simulink model "DLC_2a"  (R2023a)
settings: Solver=ode4  StartTime=0.0  StopTime=40  FixedStep=0.005  RelTol=1e-3
InitFcn:
  | DLC2
values from neighbouring files (symbols this model uses):
  K_scheduled = zeros(length(V_op), 2)    [CAL3.m]    (also in CUB.m; DLC2.m; MUS.m; OHZ.m)
  V_op = 5:5:85    [CAL3.m]    (also in CUB.m; DLC2.m; MUS.m; OHZ.m)
  X_track = [linspace(0, runway_length, 200)'; runway_length + R_track * cos(theta_circ(2:end))]    [CAL3.m]    (also in CUB.m = [0; 5000]; DLC2.m = 0:0.1:total_track_length; MUS.m = [0; 2000]; OHZ.m = [0; 2000])
  Y_track = [zeros(200, 1); R_track + R_track * sin(theta_circ(2:end))]    [CAL3.m]    (also in CUB.m = [0; 0]; DLC2.m = zeros(size(X_track)); MUS.m = [0; 0]; OHZ.m = [0; 0])
undefined symbols (not defined in the file or in its folder): planner_params, track_params, veh_params
libraries: simulink x2, slpidlib x2
(part 2 of 3)

== matlab function DLC_2a/Scopes/MATLAB Function1 ==
  settings: updateMethod=DISCRETE
  data: delta input; psi input; psi_ref input; Fx input; Fy input; Fz input; Trl input; Trr input; Tf_f input; Trl_f input; Trr_f input; w_vec input; vx input; vy input; ax input; ay input
function vehicle_frame_plotter(delta, psi, psi_ref, Fx, Fy, Fz, Trl, Trr, Tf_f, Trl_f, Trr_f, w_vec, vx, vy, ax, ay)
    coder.extrinsic('figure', 'plot', 'hold', 'axis', 'title', 'set', 'drawnow', 'patch', 'text', 'line', 'quiver', 'sprintf');
    
    persistent hWheels hSteer hSpokes hPsiRef hPsiAct hFlags hTqFlags hMotors hAxleFront hCircles hGdots hSwLabel hRwLabel hAngleLabel hVelArrow hAccArrow hVelText hAccText hCrosshairs counter
    
    if isempty(counter)
        % =====================================================================
        % STRICT CODER INITIALIZATION
        % =====================================================================
        counter = 0;
        hSteer = 0.0; hPsiRef = 0.0; hPsiAct = 0.0; hAxleFront = 0.0;
        hWheels = zeros(1,4); hFlags = zeros(1,4); hTqFlags = zeros(1,2); hMotors = zeros(1,2);
        hSpokes = zeros(1,3); hCircles = zeros(1,4); hGdots = zeros(1,4);
        hSwLabel = 0.0; hRwLabel = 0.0; hAngleLabel = 0.0;
        hVelArrow = 0.0; hAccArrow = 0.0; hVelText = 0.0; hAccText = 0.0;
        hCrosshairs = zeros(1,2);
        
        figure('Name', 'Vehicle Frame Telemetry - Car A', 'Color', 'w', 'Position', [100, 100, 750, 750]);
        hold on;
        
        % Chassis Outline & Front Axle
        plot([-1, 1, 1, -1, -1], [2, 2, -2, -2, 2], 'k', 'LineWidth', 2);
        hAxleFront = double(line([1, -1], [1.5, 1.5], 'Color', [0.2 0.2 0.2], 'LineWidth', 2));
        
        % Wheels Array Setup [FL, FR, RL, RR]
        for i = 1:4; hWheels(i) = double(patch(0, 0, [0.3 0.3 0.3])); end
        
        % =====================================================================
        % FRICTION CIRCLES, STEERING WHEEL, & YAW VECTORS
        % =====================================================================
        th_c = 0:0.1:2*pi;
        circle_x = cos(th_c); circle_y = sin(th_c);
        c_pos = [-2.0, 2.3; 2.0, 2.3; -2.0, -2.3; 2.0, -2.3]; 
        for i = 1:4
            hCircles(i) = double(plot(c_pos(i,1) + 0.5*circle_x, c_pos(i,2) + 0.5*circle_y, 'Color', [0.6 0 0.6], 'LineStyle', '--', 'LineWidth', 1.2));
            hGdots(i) = double(plot(c_pos(i,1), c_pos(i,2), 'mo', 'MarkerFaceColor', 'm', 'MarkerSize', 5));
        end
        
        hSteer = double(plot(0.4*cos(th_c), 0.4*sin(th_c) + 0.5, 'k', 'LineWidth', 3));
        hSpokes(1) = double(line([0, 0], [0.5, 0.5], 'Color', 'k', 'LineWidth', 2.5));
        hSpokes(2) = double(line([0, 0], [0.5, 0.5], 'Color', 'k', 'LineWidth', 2.5));
        hSpokes(3) = double(line([0, 0], [0.5, 0.5], 'Color', 'k', 'LineWidth', 2.5));
        
        hPsiRef = double(quiver(0, 1.8, 0, 0.8, 'r', 'LineWidth', 2.5, 'MaxHeadSize', 2));
        hPsiAct = double(quiver(0, 1.8, 0, 0.8, 'b', 'LineWidth', 2.5, 'MaxHeadSize', 2));
        
        for i = 1:4; hFlags(i) = double(text(0, 0, '', 'FontSize', 8, 'BackgroundColor', [1 1 1 0.8], 'EdgeColor', 'k')); end
        
        % =====================================================================
        % VEHICLE A POWERTRAIN GRAPHIC (Dual Motors)
        % =====================================================================
        m_b = [-.15, .15, .15, -.15]; m_w = [.2, .2, -.2, -.2];
        hMotors(1) = double(patch(m_b - 0.6, m_w - 1.5, [0.5 0.5 0.5])); % Left Motor
        hMotors(2) = double(patch(m_b + 0.6, m_w - 1.5, [0.5 0.5 0.5])); % Right Motor
        
        hTqFlags(1) = double(text(-0.6, -0.9, '', 'FontSize', 10, 'FontWeight', 'bold', 'HorizontalAlignment', 'center'));
        hTqFlags(2) = double(text(0.6, -0.9, '', 'FontSize', 10, 'FontWeight', 'bold', 'HorizontalAlignment', 'center'));
        
        % Labels
        hSwLabel = double(text(0, 1.2, '', 'FontSize', 9, 'FontWeight', 'bold', 'HorizontalAlignment', 'center'));
        hRwLabel = double(text(0, 1.65, '', 'FontSize', 9, 'FontWeight', 'bold', 'HorizontalAlignment', 'center', 'Color', [0 0.5 0]));
        hAngleLabel = double(text(0, 2.8, '', 'FontSize', 10, 'FontWeight', 'bold', 'HorizontalAlignment', 'center', 'Color', [0.4 0 0.6]));

        % =====================================================================
        % SHARED-ORIGIN VELOCITY & ACCELERATION VECTORS
        % =====================================================================
        hCrosshairs(1) = double(plot([-2.0 2.0], [-3.8 -3.8], 'k:', 'Color', [0.7 0.7 0.7]));
        hCrosshairs(2) = double(plot([0 0], [-4.2 -1.8], 'k:', 'Color', [0.7 0.7 0.7]));

        hVelArrow = double(quiver(0, -3.8, 0, 0, 'Color', [0 0.4 0.8], 'LineWidth', 2.5, 'MaxHeadSize', 2, 'AutoScale', 'off'));
        hAccArrow = double(quiver(0, -3.8, 0, 0, 'Color', [0.8 0.3 0], 'LineWidth', 2.5, 'MaxHeadSize', 2, 'AutoScale', 'off'));

        hVelText = double(text(-2.0, -4.3, '', 'FontSize', 9, 'FontWeight', 'bold', 'HorizontalAlignment', 'center', 'Color', [0 0.4 0.8]));
        hAccText = double(text(2.0, -4.3, '', 'FontSize', 9, 'FontWeight', 'bold', 'HorizontalAlignment', 'center', 'Color', [0.8 0.3 0]));
        
        axis([-4.5 4.5 -4.5 4.5]); axis equal; grid on;
        title('Dynamics - Car A (Dual Motor): Forces & Friction Circles');
    end
    counter = counter + 1;
    
    % --- UPDATE LOOP ---
    if mod(counter, 10) == 0
        R_delta = [cos(delta) -sin(delta); sin(delta) cos(delta)];
        w_orig = [-.2 .2 .2 -.2; .4 .4 -.4 -.4]; 
        w_rot = R_delta * w_orig;
        
        set(hWheels(1), 'XData', w_rot(1,:) - 1, 'YData', w_rot(2,:) + 1.5); 
        set(hWheels(2), 'XData', w_rot(1,:) + 1, 'YData', w_rot(2,:) + 1.5); 
        set(hWheels(3), 'XData', w_orig(1,:) - 1, 'YData', w_orig(2,:) - 1.5); 
        set(hWheels(4), 'XData', w_orig(1,:) + 1, 'YData', w_orig(2,:) - 1.5); 
        
        set(hAxleFront, 'XData', [mean(w_rot(1,:) - 1), mean(w_rot(1,:) + 1)], 'YData', [mean(w_rot(2,:) + 1.5), mean(w_rot(2,:) + 1.5)]);
        
        sw_a = delta * 14; 
        th_sw = (0:0.1:2*pi) + sw_a;
        set(hSteer, 'XData', 0.4*cos(th_sw), 'YData', 0.4*sin(th_sw) + 0.5);
        spk = [0, pi, 1.5*pi] + sw_a;
        for j=1:3; set(hSpokes(j), 'XData', [0, 0.4*cos(spk(j))], 'YData', [0.5, 0.5 + 0.4*sin(spk(j))]); end
        
        set(hSwLabel, 'String', sprintf('SW: %.1f deg', sw_a * 180/pi));
        set(hRwLabel, 'String', sprintf('RW: %.1f deg', delta * 180/pi));
        
        psi_e = psi_ref - psi; 
        set(hPsiRef, 'UData', 0.8*sin(psi_e), 'VData', 0.8*cos(psi_e));
        set(hPsiAct, 'UData', 0, 'VData', 0.8);
        set(hAngleLabel, 'String', sprintf('Sideslip: %.1f deg', psi_e * 180/pi));
        
        fb = [abs(Tf_f/2), abs(Tf_f/2), abs(Trl_f), abs(Trr_f)]; 
        mu = 1.0;
        c_pos = [-2.0, 2.3; 2.0, 2.3; -2.0, -2.3; 2.0, -2.3]; 
        th_c = 0:0.1:2*pi;
        rpm_vec = w_vec * (30 / pi);
        
        for i = 1:4
            if fb(i) > 5; set(hWheels(i), 'FaceColor', [0.8 0 0]); else set(hWheels(i), 'FaceColor', [0.3 0.3 0.3]); end
            F_max = max(100, mu * Fz(i));
            scale = 0.5 / 6000; 
            set(hCircles(i), 'XData', c_pos(i,1) + F_max*scale*cos(th_c), 'YData', c_pos(i,2) + F_max*scale*sin(th_c));
            set(hGdots(i), 'XData', c_pos(i,1) + Fy(i)*scale, 'YData', c_pos(i,2) + Fx(i)*scale);
        end
        
        % Dual Motor Visualization Logic
        mt = [Trl, Trr]; 
        for k = 1:2
            if mt(k) > 0.1; set(hMotors(k), 'FaceColor', [0 0.7 0]); 
            elseif mt(k) < -0.1; set(hMotors(k), 'FaceColor', [0.7 0 0]); 
            else set(hMotors(k), 'FaceColor', [0.5 0.5 0.5]); end
            
            set(hTqFlags(k), 'String', sprintf('%.1f Nm', mt(k)));
        end
        
        pos = [-4.1, 1.5; 2.8, 1.5; -4.1, -1.5; 2.8, -1.5]; 
        for i = 1:4
            f_str = sprintf('Fx: %.0f\nFy: %.0f\nFz: %.0f\nFric: %.1f\nRPM: %.0f', Fx(i), Fy(i), Fz(i), fb(i), rpm_vec(i));
            set(hFlags(i), 'Position', [pos(i,1), pos(i,2)], 'String', f_str);
        end

        % =====================================================================
        % UPDATE DYNAMIC VECTORS
        % =====================================================================
        vx_kmh = vx * 3.6;
        vy_kmh = vy * 3.6;
        ax_g = ax / 9.81;
        ay_g = ay / 9.81;

        vel_scale = 0.015; 
        acc_scale = 0.8;   

        set(hVelArrow, 'UData', -vy_kmh * vel_scale, 'VData', vx_kmh * vel_scale);
        set(hAccArrow, 'UData', -ay_g * acc_scale, 'VData', ax_g * acc_scale);

        set(hVelText, 'String', sprintf('Vx: %.1f | Vy: %.1f\n[km/h]', vx_kmh, vy_kmh));
        set(hAccText, 'String', sprintf('Ax: %.2f | Ay: %.2f\n[G]', ax_g, ay_g));
        
        drawnow limitrate;
    end
end

== matlab function DLC_2a/Vehicle & Powertrain Plant1/MATLAB Function ==
  data: delta input; Trr_m input; Trl_m input; Trr_f input; Trl_f input; Tf_f input; vx input; vy input; r input; psi input; SOC input; T_batt input; T_motor input; w_fl input; w_fr input; w_rl input; w_rr input; vx_dot output; vy_dot output; r_dot output; X_dot output; Y_dot output; psi_dot output; s_dot output; SOC_dot output; T_batt_dot output; T_mot_dot output; Fz_f_tot output; Fz_r_tot output; Fz_rl output; Fz_rr output; Fx_vec output; Fy_vec output; Fz_vec output; w_vec output; w_dot_vec output; veh_params parameter
function [vx_dot, vy_dot, r_dot, X_dot, Y_dot, psi_dot, s_dot, SOC_dot, T_batt_dot, T_mot_dot, Fz_f_tot, Fz_r_tot, Fz_rl, Fz_rr, Fx_vec, Fy_vec, Fz_vec, w_vec, w_dot_vec] = vehicle_physics_engine(delta, Trr_m, Trl_m, Trr_f, Trl_f, Tf_f, vx, vy, r, psi, SOC, T_batt, T_motor, w_fl, w_fr, w_rl, w_rr, veh_params)
    % =========================================================================
    % HIGH-FIDELITY EV VEHICLE DYNAMICS PLANT MODEL (ANTI-SINGULARITY PATCHED)
    % =========================================================================
    
    % ---------------------------------------------------------------------
    % 1. UNPACK CENTRALIZED PARAMETERS
    % ---------------------------------------------------------------------
    m = veh_params.m; Iz = veh_params.Iz; lf = veh_params.lf; lr = veh_params.lr; L = veh_params.L;
    tw = veh_params.tw; h_cg = veh_params.h_cg; Rw = veh_params.Rw; Iw = veh_params.Iw; 
    G = veh_params.G; g = veh_params.g; rho = veh_params.rho; CdA = veh_params.CdA;
    roll_bias_f = veh_params.roll_bias_f; 
    
    mu_max = veh_params.mu_max; C_rr = veh_params.C_rr;
    ks_f = veh_params.ks_f; ks_r = veh_params.ks_r;
    C_tire = veh_params.C_tire; E_tire = veh_params.E_tire;
    
    if abs(vx) < 0.5
        vx_safe = 0.5 * sign(vx + 1e-6); % Prevents absolute zero, preserves direction
    else
        vx_safe = vx;
    end
    
    % FIX 1: Preserved-Sign Aerodynamic Drag
    % vx_safe * abs(vx_safe) ensures drag always pushes AGAINST the car, even in reverse.
    F_aero_drag = 0.5 * rho * CdA * vx_safe * abs(vx_safe);

    % ---------------------------------------------------------------------
    % 2. DYNAMIC TIRE PEAK CALIBRATION
    % ---------------------------------------------------------------------
    Fz_axle_f_static = m * g * (lr / L); 
    Fz_axle_r_static = m * g * (lf / L); 
    
    D_tire_f = mu_max * (Fz_axle_f_static / 2); 
    D_tire_r = mu_max * (Fz_axle_r_static / 2); 
    
    B_tire_f = ks_f / (C_tire * D_tire_f * 2); 
    B_tire_r = ks_r / (C_tire * D_tire_r * 2); 
    
    % ---------------------------------------------------------------------
    % 3. 3D WEIGHT TRANSFER (WITH SUSPENSION CAPS)
    % ---------------------------------------------------------------------
    Trr_tot = Trr_m * G + Trr_f;
    Trl_tot = Trl_m * G + Trl_f;
    Tf_tot_half = Tf_f / 2; 
    
    Fx_fl_tq = Tf_tot_half / Rw; Fx_fr_tq = Tf_tot_half / Rw;
    Fx_rl_tq = Trl_tot / Rw; Fx_rr_tq = Trr_tot / Rw;
    
    % Using corrected aero drag
    ax_est = ((Fx_fl_tq + Fx_fr_tq + Fx_rl_tq + Fx_rr_tq) - F_aero_drag) / m;
    ay_est = vx_safe * r;
    
    Fz_f_tot = m * g * (lr / L) - m * ax_est * (h_cg / L);
    Fz_r_tot = m * g * (lf / L) + m * ax_est * (h_cg / L);
    
    dFz_y_f = m * ay_est * (h_cg / tw) * roll_bias_f;
    dFz_y_r = m * ay_est * (h_cg / tw) * (1 - roll_bias_f);
    
    % FIX 2: Suspension Caps. Prevents Fz from exceeding physical limits in a spin
    Fz_max_f = Fz_axle_f_static * 2.5; 
    Fz_max_r = Fz_axle_r_static * 2.5;
    
    Fz_fl = max(100, min(Fz_max_f, Fz_f_tot / 2 + dFz_y_f));
    Fz_fr = max(100, min(Fz_max_f, Fz_f_tot / 2 - dFz_y_f));
    Fz_rl = max(100, min(Fz_max_r, Fz_r_tot / 2 + dFz_y_r));
    Fz_rr = max(100, min(Fz_max_r, Fz_r_tot / 2 - dFz_y_r));
    Fz_vec = [Fz_fl, Fz_fr, Fz_rl, Fz_rr];
    
    % ---------------------------------------------------------------------
    % 4. VECTOR-SUM PACEJKA COMBINED SLIP MODEL
    % ---------------------------------------------------------------------
    v_hub_fl = vx_safe - (tw / 2) * r; v_hub_fr = vx_safe + (tw / 2) * r;
    v_hub_rl = vx_safe - (tw / 2) * r; v_hub_rr = vx_safe + (tw / 2) * r;
    
    k_fl = (w_fl * Rw - v_hub_fl) / max(abs(v_hub_fl), 1.0);
    k_fr = (w_fr * Rw - v_hub_fr) / max(abs(v_hub_fr), 1.0);
    k_rl = (w_rl * Rw - v_hub_rl) / max(abs(v_hub_rl), 1.0);
    k_rr = (w_rr * Rw - v_hub_rr) / max(abs(v_hub_rr), 1.0);
    
    % FIX 3: Absolute value on denomiator prevents inverted slip angles in reverse
    alpha_fl = delta - atan((vy + lf * r) / max(abs(v_hub_fl), 1.0));
    alpha_fr = delta - atan((vy + lf * r) / max(abs(v_hub_fr), 1.0));
    alpha_rl = -atan((vy - lr * r) / max(abs(v_hub_rl), 1.0));
    alpha_rr = -atan((vy - lr * r) / max(abs(v_hub_rr), 1.0));
    
    sigma_fl = sqrt(k_fl^2 + tan(alpha_fl)^2) + 1e-6;
    sigma_fr = sqrt(k_fr^2 + tan(alpha_fr)^2) + 1e-6;
    sigma_rl = sqrt(k_rl^2 + tan(alpha_rl)^2) + 1e-6;
    sigma_rr = sqrt(k_rr^2 + tan(alpha_rr)^2) + 1e-6;
    
    F_tot_fl = mu_max * Fz_fl * sin(C_tire * atan(B_tire_f * sigma_fl - E_tire * (B_tire_f * sigma_fl - atan(B_tire_f * sigma_fl))));
    F_tot_fr = mu_max * Fz_fr * sin(C_tire * atan(B_tire_f * sigma_fr - E_tire * (B_tire_f * sigma_fr - atan(B_tire_f * sigma_fr))));
    F_tot_rl = mu_max * Fz_rl * sin(C_tire * atan(B_tire_r * sigma_rl - E_tire * (B_tire_r * sigma_rl - atan(B_tire_r * sigma_rl))));
    F_tot_rr = mu_max * Fz_rr * sin(C_tire * atan(B_tire_r * sigma_rr - E_tire * (B_tire_r * sigma_rr - atan(B_tire_r * sigma_rr))));
    
    Fx_fl = F_tot_fl * (k_fl / sigma_fl) - C_rr * Fz_fl * tanh(v_hub_fl * 10);
    Fx_fr = F_tot_fr * (k_fr / sigma_fr) - C_rr * Fz_fr * tanh(v_hub_fr * 10);
    Fx_rl = F_tot_rl * (k_rl / sigma_rl) - C_rr * Fz_rl * tanh(v_hub_rl * 10);
    Fx_rr = F_tot_rr * (k_rr / sigma_rr) - C_rr * Fz_rr * tanh(v_hub_rr * 10);
    Fx_vec = [Fx_fl, Fx_fr, Fx_rl, Fx_rr];
    
    Fy_fl = F_tot_fl * (tan(alpha_fl) / sigma_fl);
    Fy_fr = F_tot_fr * (tan(alpha_fr) / sigma_fr);
    Fy_rl = F_tot_rl * (tan(alpha_rl) / sigma_rl);
    Fy_rr = F_tot_rr * (tan(alpha_rr) / sigma_rr);
    Fy_vec = [Fy_fl, Fy_fr, Fy_rl, Fy_rr];
    
    % ---------------------------------------------------------------------
    % 5. CHASSIS & WHEEL INTEGRATORS
    % ---------------------------------------------------------------------
    w_fl_dot = (-abs(Tf_f / 2) * sign(w_fl) - Fx_fl * Rw) / Iw;
    w_fr_dot = (-abs(Tf_f / 2) * sign(w_fr) - Fx_fr * Rw) / Iw;
    w_rl_dot = (Trl_m * G - abs(Trl_f) * sign(w_rl) - Fx_rl * Rw) / Iw;
    w_rr_dot = (Trr_m * G - abs(Trr_f) * sign(w_rr) - Fx_rr * Rw) / Iw;
    w_dot_vec = [w_fl_dot, w_fr_dot, w_rl_dot, w_rr_dot];
    w_vec = [w_fl, w_fr, w_rl, w_rr];
    
    sum_Fx = (Fx_fl + Fx_fr) * cos(delta) - (Fy_fl + Fy_fr) * sin(delta) + Fx_rl + Fx_rr;
    vx_dot = (sum_Fx - F_aero_drag) / m + vy * r;
    
    sum_Fy = (Fy_fl + Fy_fr) * cos(delta) + (Fx_fl + Fx_fr) * sin(delta) + Fy_rl + Fy_rr;
    vy_dot = sum_Fy / m - vx_safe * r;
    
    M_front = lf * ((Fy_fl + Fy_fr) * cos(delta) + (Fx_fl + Fx_fr) * sin(delta));
    M_rear  = -lr * (Fy_rl + Fy_rr);
    M_tv    = (Fx_rr - Fx_rl) * (tw / 2); 
    r_dot  = (M_front + M_rear + M_tv) / Iz;
    
    X_dot   = vx_safe * cos(psi) - vy * sin(psi);
    Y_dot   = vx_safe * sin(psi) + vy * cos(psi);
    psi_dot = r;
    s_dot   = vx_safe;
    
    % ---------------------------------------------------------------------
    % 6. THERMALS & SOC
    % ---------------------------------------------------------------------
    P_mech = (Trr_m + Trl_m) * G * (vx_safe / Rw);
    P_elec = P_mech; 
    
    if P_mech > 500
        P_elec = P_mech / 0.90; 
    elseif P_mech < -500
        P_elec = P_mech * 0.90; 
    end
    
    I_curr = P_elec / veh_params.V_pack;
    SOC_dot = -I_curr / (veh_params.Cap_Ah * 3600);
    
    T_batt_dot = ((I_curr^2) * veh_params.R_pack - veh_params.hA_cool_batt * (T_batt - veh_params.T_coolant_batt)) / (veh_params.m_batt * veh_params.cp_batt);
    T_mot_dot  = (abs(P_elec - P_mech) - veh_params.hA_cool_motor * (T_motor - veh_params.T_ambient)) / (veh_params.m_motor * veh_params.cp_motor);
end

== matlab function DLC_2a/Vehicle Control Unit (VCU)1/MATLAB Function ==
  data: delta_curr input; pedal input; T_rr_motor_raw output; vx_curr input; vy_curr input; r_curr input; kappa_ref input; Fz_f_total input; Fz_r_total input; Fz_rl input; Fz_rr input; SOC input; T_batt input; T_motor input; V_op parameter; K_scheduled parameter; T_rl_motor_raw output; T_rr_fric output; w_vec input; T_rl_fric output; T_f_fric output; Mz_cmd output; r_ref output
function [T_rr_motor_raw, T_rl_motor_raw, T_rr_fric, T_rl_fric, T_f_fric, Mz_cmd, r_ref] = vcu_allocator(delta_curr, pedal, vx_curr, vy_curr, r_curr, kappa_ref, Fz_f_total, Fz_r_total, Fz_rl, Fz_rr, SOC, T_batt, T_motor, V_op, K_scheduled, w_vec)
    
    T_rr_motor_raw = 0.0;
    T_rl_motor_raw = 0.0;
    T_rr_fric = 0.0;
    T_rl_fric = 0.0;
    T_f_fric = 0.0;
    Mz_cmd = 0.0;
    Rw = 0.34; tw = 1.65; G = 10; mu_max = 1.2;
    
    % --- Per-Motor Limits (Total System = 500 kW, 800 Nm) ---
    P_motor_base = 250000; % 250 kW per motor 
    T_motor_max = 400;     % 400 Nm per motor 
    T_fric_max_per_wheel = 3500;
    % --------------------------------------------------------
    
    % --- Battery and Thermal Derating ---
    T_batt_cal = [-10, 0, 15, 45, 55, 60]; P_derate_batt_cal = [0, 0.5, 1.0, 1.0, 0.2, 0];
    T_motor_cal = [30, 90, 110, 130, 150]; P_derate_motor_cal = [1.0, 1.0, 0.8, 0.2, 0];
    SOC_vec = [0, 0.05, 0.15, 0.85, 0.95, 1.0]; 
    P_derate_SOC_dis = [0, 0.1, 1.0, 1.0, 1.0, 1.0]; P_derate_SOC_chg = [1.0, 1.0, 1.0, 1.0, 0.1, 0];
    
    derate_T_batt = interp1(T_batt_cal, P_derate_batt_cal, T_batt(1), 'linear', 0);
    derate_T_mot  = interp1(T_motor_cal, P_derate_motor_cal, T_motor(1), 'linear', 0);
    derate_T_total = min(derate_T_batt, derate_T_mot);
    
    derate_S_dis = interp1(SOC_vec, P_derate_SOC_dis, SOC(1), 'linear', 0);
    derate_S_chg = interp1(SOC_vec, P_derate_SOC_chg, SOC(1), 'linear', 0);
    
    P_avail_dis = P_motor_base * min(derate_T_total, derate_S_dis);
    P_avail_chg = P_motor_base * min(derate_T_total, derate_S_chg);
    
    vx_lqr = max(vx_curr(1), 5.0);
    
    % --- Speed-based Torque Vectoring Blending (45 km/h to 50 km/h) ---
    vx_kmh = vx_curr(1) * 3.6;
    tv_blend_lower = 45.0; 
    tv_blend_upper = 50.0; 
    
    if vx_kmh >= tv_blend_upper
        tv_blend = 1.0;
    elseif vx_kmh <= tv_blend_lower
        tv_blend = 0.0;
    else
        tv_blend = (vx_kmh - tv_blend_lower) / (tv_blend_upper - tv_blend_lower);
    end
    
    % --- LQR Yaw Moment Calculation ---
    K_dyn_1 = interp1(V_op, K_scheduled(:,1), vx_lqr, 'linear', 'extrap');
    K_dyn_2 = interp1(V_op, K_scheduled(:,2), vx_lqr, 'linear', 'extrap');
             
    % Dynamic Ackermann Reference
    L = 2.6; % Wheelbase
    K_us = 0.002; % Small understeer gradient (optional)
    r_ref = (vx_lqr * delta_curr(1)) / (L * (1 + K_us * vx_lqr^2));
    
    Mz_req = tv_blend * -(K_dyn_1(1) * vy_curr(1) + K_dyn_2(1) * (r_curr(1) - r_ref));
    Mz_cmd = max(-2500, min(2500, Mz_req)); 
    
    T_delta_wheel_raw = max(-1500, min(1500, (Mz_cmd * Rw) / tw));
    
    % =========================================================================
    % --- DYNAMIC MOTOR POWER LIMITS (Hyperbolic Torque Derating) ---
    % =========================================================================
    % Calculate actual motor speed from wheel speed (rad/s)
    % w_vec = [w_fl, w_fr, w_rl, w_rr]
    w_motor_rl = max(abs(w_vec(3) * G), 0.1); % Prevent div-by-zero at standstill
    w_motor_rr = max(abs(w_vec(4) * G), 0.1); 
    
    % Power-limited torque curve: T_max = P_max / w
    T_limit_rl_dis = P_avail_dis / w_motor_rl;
    T_limit_rr_dis = P_avail_dis / w_motor_rr;
    T_limit_rl_chg = P_avail_chg / w_motor_rl;
    T_limit_rr_chg = P_avail_chg / w_motor_rr;
    
    % Final motor bounds (Minimum of Inverter current limit and Power limit)
    T_motor_lim_rl_dis = min(T_motor_max, T_limit_rl_dis);
    T_motor_lim_rr_dis = min(T_motor_max, T_limit_rr_dis);
    
    T_motor_lim_rl_chg = max(-T_motor_max, -T_limit_rl_chg);
    T_motor_lim_rr_chg = max(-T_motor_max, -T_limit_rr_chg);
    % =========================================================================
    
    T_grip_lim_rl_wheel = mu_max * Fz_rl(1) * Rw * 0.90; 
    T_grip_lim_rr_wheel = mu_max * Fz_rr(1) * Rw * 0.90;
    
    % Combine physical motor limits with dynamic grip limits
    T_max_rl_motor = min(T_motor_lim_rl_dis, T_grip_lim_rl_wheel / G);
    T_max_rr_motor = min(T_motor_lim_rr_dis, T_grip_lim_rr_wheel / G);
    T_min_rl_motor = max(T_motor_lim_rl_chg, -T_grip_lim_rl_wheel / G);
    T_min_rr_motor = max(T_motor_lim_rr_chg, -T_grip_lim_rr_wheel / G);
    
    weight_rl = Fz_rl(1) / max(1, (Fz_rl(1) + Fz_rr(1))); 
    weight_rr = Fz_rr(1) / max(1, (Fz_rl(1) + Fz_rr(1)));
    
    % --- DRIVE MODE ---
    if pedal(1) >= 0
        % Total requested drive torque, limited by combined max capabilities
        T_req_total_motor = pedal(1) * (T_max_rl_motor + T_max_rr_motor); 
        
        T_rr_base_motor = T_req_total_motor * weight_rr;
        T_rl_base_motor = T_req_total_motor * weight_rl; 
        
        T_rr_ideal = max(T_min_rr_motor, min(T_max_rr_motor, T_rr_base_motor + (T_delta_wheel_raw/G)));
        T_rl_ideal = max(T_min_rl_motor, min(T_max_rl_motor, T_rl_base_motor - (T_delta_wheel_raw/G)));
        
        % Traction Control (TCS)
        v_hub_rl = max(vx_curr(1) - (tw/2)*r_curr(1), 1.0);
        v_hub_rr = max(vx_curr(1) + (tw/2)*r_curr(1), 1.0);
        
        kappa_rl = (w_vec(3)*Rw - v_hub_rl) / v_hub_rl;
        kappa_rr = (w_vec(4)*Rw - v_hub_rr) / v_hub_rr;
        
        slip_target = 0.10;
        Kp_tcs = 1000;
        
        if kappa_rl > slip_target
            T_rl_ideal = max(0, T_rl_ideal - Kp_tcs * (kappa_rl - slip_target));
        end
        if kappa_rr > slip_target
            T_rr_ideal = max(0, T_rr_ideal - Kp_tcs * (kappa_rr - slip_target));
        end
        
        T_rr_fric = 0; T_rl_fric = 0; T_f_fric = 0;
        
    % --- BRAKE MODE ---
    else
        bias_f = 0.70;
        total_grip_cap_wheel = mu_max * (Fz_f_total(1) + Fz_r_total(1)) * Rw * 0.90;
        T_req_total_wheel = pedal(1) * total_grip_cap_wheel; 
        
        T_req_front_wheel = T_req_total_wheel * bias_f; 
        T_req_rear_wheel = T_req_total_wheel * (1 - bias_f);
        
        T_f_fric = max(-mu_max * Fz_f_total(1) * Rw * 0.90, T_req_front_wheel);
        
        T_base_rr = max(-(T_grip_lim_rr_wheel - abs(T_delta_wheel_raw)), T_req_rear_wheel * weight_rr);
        T_base_rl = max(-(T_grip_lim_rl_wheel - abs(T_delta_wheel_raw)), T_req_rear_wheel * weight_rl);
        
        T_rr_ideal_wheel = T_base_rr + T_delta_wheel_raw; 
        T_rl_ideal_wheel = T_base_rl - T_delta_wheel_raw;
        
        % Anti-Lock Braking (ABS)
        v_hub_fl = max(vx_curr(1) - (tw/2)*r_curr(1), 1.0);
        v_hub_fr = max(vx_curr(1) + (tw/2)*r_curr(1), 1.0);
        v_hub_rl = max(vx_curr(1) - (tw/2)*r_curr(1), 1.0);
        v_hub_rr = max(vx_curr(1) + (tw/2)*r_curr(1), 1.0);
        
        kappa_fl = (w_vec(1)*Rw - v_hub_fl) / v_hub_fl;
        kappa_fr = (w_vec(2)*Rw - v_hub_fr) / v_hub_fr;
        kappa_rl = (w_vec(3)*Rw - v_hub_rl) / v_hub_rl;
        kappa_rr = (w_vec(4)*Rw - v_hub_rr) / v_hub_rr;
        
        slip_limit_abs = -0.10;
        Kp_abs = 5000;
        
        worst_kappa_f = min(kappa_fl, kappa_fr);
        if worst_kappa_f < slip_limit_abs
            T_f_fric = min(0, T_f_fric - Kp_abs * (worst_kappa_f - slip_limit_abs));
        end
        if kappa_rl < slip_limit_abs
            T_rl_ideal_wheel = min(0, T_rl_ideal_wheel - Kp_abs * (kappa_rl - slip_limit_abs));
        end
        if kappa_rr < slip_limit_abs
            T_rr_ideal_wheel = min(0, T_rr_ideal_wheel - Kp_abs * (kappa_rr - slip_limit_abs));
        end
        
        T_rr_ideal = max(T_min_rr_motor, min(T_max_rr_motor, T_rr_ideal_wheel / G));
        T_rl_ideal = max(T_min_rl_motor, min(T_max_rl_motor, T_rl_ideal_wheel / G));
        
        T_rr_fric = max(-T_fric_max_per_wheel, min(0, T_rr_ideal_wheel - (T_rr_ideal * G)));
        T_rl_fric = max(-T_fric_max_per_wheel, min(0, T_rl_ideal_wheel - (T_rl_ideal * G)));
        
        if vx_curr(1) < 2.0
            T_f_fric = 0; T_rr_fric = 0; T_rl_fric = 0;
            T_rr_ideal = 0; T_rl_ideal = 0;
        end
    end
    
    T_rr_motor_raw = T_rr_ideal;
    T_rl_motor_raw = T_rl_ideal;
end

== matlab function DLC_2a/Scopes1/MATLAB Function ==
  settings: updateMethod=DISCRETE
  data: X_curr input; Y_curr input; psi_curr input; vx_curr input; delta_curr input; t_curr input; X_track parameter; Y_track parameter
function live_track_plotter(X_curr, Y_curr, psi_curr, vx_curr, delta_curr, t_curr, X_track, Y_track)
    coder.extrinsic('figure', 'plot', 'hold', 'axis', 'title', 'xlabel', 'ylabel', 'set', 'drawnow', 'animatedline', 'addpoints', 'legend', 'grid', 'patch', 'text');
    
    persistent hFig hCar hTrail hText counter 
    persistent hTimer1 hTimer2 hTimer3 hTimer4 hTimer5
    persistent lap_count lap_start_time lap_trigger_ready
    persistent past_lap_1 past_lap_2 past_lap_3 past_lap_4 past_lap_5
    
    if isempty(counter)
        counter = 0;
        lap_count = 1;
        lap_start_time = 0;
        lap_trigger_ready = false;
        
        past_lap_1 = 0; past_lap_2 = 0; past_lap_3 = 0; past_lap_4 = 0; past_lap_5 = 0;
        
        hFig = figure('Name', 'Live Telemetry: Silverstone / DLC', 'Color', 'w', 'Position', [100, 100, 800, 600]);
        plot(X_track, Y_track, '--', 'Color', [0.4 0.4 0.4], 'LineWidth', 1.5); hold on;
        
        plot(X_track(1), Y_track(1), 'ko', 'MarkerSize', 10, 'MarkerFaceColor', 'g', 'LineWidth', 1.5);
        text(X_track(1) - 50, Y_track(1) + 70, 'Start / Finish', 'FontSize', 10, 'FontWeight', 'bold', 'Color', 'k', 'BackgroundColor', [1 1 1 0.7]);
        
        hTrail = animatedline('Color', 'b', 'LineWidth', 1.5);
        
        hCar = patch(0, 0, [0.8 0 0], 'EdgeColor', 'k', 'LineWidth', 1);
        set(hCar, 'FaceAlpha', 0.8); 
        
        hText = text(0, 0, ' Init...', 'FontSize', 10, 'FontWeight', 'bold', 'BackgroundColor', [1 1 1 0.8], 'EdgeColor', 'k', 'Margin', 2);
        
        box_props = {'Units', 'normalized', 'HorizontalAlignment', 'right', 'FontSize', 12, 'FontWeight', 'bold', 'BackgroundColor', [1 1 1 0.9], 'EdgeColor', 'k', 'Margin', 4, 'Visible', 'off'};
        
        hTimer1 = text(0.95, 0.95, '', box_props{:});
        hTimer2 = text(0.95, 0.89, '', box_props{:});
        hTimer3 = text(0.95, 0.83, '', box_props{:});
        hTimer4 = text(0.95, 0.77, '', box_props{:});
        hTimer5 = text(0.95, 0.71, '', box_props{:});
        
        axis equal; grid on;
        title('Live Vehicle Tracking with Telemetry');
        xlabel('X Position (meters)'); ylabel('Y Position (meters)');
        legend('Reference Track', 'Start/Finish', 'Driven Path', 'EV Position & Heading', 'Telemetry', 'Location', 'best');
    end
    counter = counter + 1;
    
    dist_to_origin = sqrt((X_curr - X_track(1))^2 + (Y_curr - Y_track(1))^2);
    
    if dist_to_origin > 50
        lap_trigger_ready = true;
    end
    
    if lap_trigger_ready && dist_to_origin < 15
        completed_lap_time = t_curr - lap_start_time;
        if lap_count == 1
            past_lap_1 = completed_lap_time;
        elseif lap_count == 2
            past_lap_2 = completed_lap_time;
        elseif lap_count == 3
            past_lap_3 = completed_lap_time;
        elseif lap_count == 4
            past_lap_4 = completed_lap_time;
        elseif lap_count == 5
            past_lap_5 = completed_lap_time;
        end
        
        lap_count = lap_count + 1;
        lap_start_time = t_curr;
        lap_trigger_ready = false; 
    end
    
    if mod(counter, 10) == 0
        addpoints(hTrail, X_curr, Y_curr);
        
        % --- REALISTIC 1:1 VEHICLE SCALING ---
        L_vis = 4.5; % 4.5 meters long
        W_vis = 1.9; % 1.9 meters wide
        % ------------------------------------
        
        base_X = [L_vis/2,  L_vis*0.3,   0,       -L_vis*0.35, -L_vis/2,  -L_vis/2,   -L_vis*0.35,  0,        L_vis*0.3,   L_vis/2];
        base_Y = [0,        W_vis*0.45, W_vis/2,  W_vis/2,     W_vis*0.3, -W_vis*0.3, -W_vis/2,    -W_vis/2, -W_vis*0.45, 0];
        
        R = [cos(psi_curr), -sin(psi_curr); 
             sin(psi_curr),  cos(psi_curr)];
             
        rotated_coords = R * [base_X; base_Y];
        final_X = rotated_coords(1, :) + X_curr;
        final_Y = rotated_coords(2, :) + Y_curr;
        
        set(hCar, 'XData', final_X, 'YData', final_Y);
        
        speed_kmh = vx_curr * 3.6;
        steer_deg = delta_curr * (180 / pi);
        
        telemetry_str = sprintf(' Spd: %.1f km/h\n Steer. Ang.: %.1f deg', speed_kmh, steer_deg);
        
        % Brought the text box much closer to the scaled vehicle
        set(hText, 'Position', [X_curr + 10, Y_curr + 10], 'String', telemetry_str);
        
        current_live_time = t_curr - lap_start_time;
        
        if lap_count == 1
            set(hTimer1, 'String', sprintf(' Lap 1: %d:%06.3f (Live) ', int32(floor(current_live_time/60)), mod(current_live_time, 60)), 'Visible', 'on');
        elseif lap_count > 1
            set(hTimer1, 'String', sprintf(' Lap 1: %d:%06.3f ', int32(floor(past_lap_1/60)), mod(past_lap_1, 60)), 'Visible', 'on');
        end
        
        if lap_count == 2
            set(hTimer2, 'String', sprintf(' Lap 2: %d:%06.3f (Live) ', int32(floor(current_live_time/60)), mod(current_live_time, 60)), 'Visible', 'on');
        elseif lap_count > 2
            set(hTimer2, 'String', sprintf(' Lap 2: %d:%06.3f ', int32(floor(past_lap_2/60)), mod(past_lap_2, 60)), 'Visible', 'on');
        end
        
        if lap_count == 3
            set(hTimer3, 'String', sprintf(' Lap 3: %d:%06.3f (Live) ', int32(floor(current_live_time/60)), mod(current_live_time, 60)), 'Visible', 'on');
        elseif lap_count > 3
            set(hTimer3, 'String', sprintf(' Lap 3: %d:%06.3f ', int32(floor(past_lap_3/60)), mod(past_lap_3, 60)), 'Visible', 'on');
        end
        
        if lap_count == 4
            set(hTimer4, 'String', sprintf(' Lap 4: %d:%06.3f (Live) ', int32(floor(current_live_time/60)), mod(current_live_time, 60)), 'Visible', 'on');
        elseif lap_count > 4
            set(hTimer4, 'String', sprintf(' Lap 4: %d:%06.3f ', int32(floor(past_lap_4/60)), mod(past_lap_4, 60)), 'Visible', 'on');
        end
        
        if lap_count == 5
            set(hTimer5, 'String', sprintf(' Lap 5: %d:%06.3f (Live) ', int32(floor(current_live_time/60)), mod(current_live_time, 60)), 'Visible', 'on');
        elseif lap_count > 5
            set(hTimer5, 'String', sprintf(' Lap 5: %d:%06.3f ', int32(floor(past_lap_5/60)), mod(past_lap_5, 60)), 'Visible', 'on');
        end
        
        drawnow limitrate; 
    end
end

== matlab function DLC_2a/Scopes1/MATLAB Function1 ==
  settings: updateMethod=DISCRETE
  data: delta input; psi input; psi_ref input; Fx input; Fy input; Fz input; Trl input; Trr input; Tf_f input; Trl_f input; Trr_f input; w_vec input
function vehicle_frame_plotter(delta, psi, psi_ref, Fx, Fy, Fz, Trl, Trr, Tf_f, Trl_f, Trr_f, w_vec)
    coder.extrinsic('figure', 'plot', 'hold', 'axis', 'title', 'set', 'drawnow', 'patch', 'text', 'line', 'quiver', 'sprintf');
    
    persistent hFig hWheels hSteer hSpokes hPsiRef hPsiAct hFlags hTqFlags hMotors hAxle hCircles hGdots hSwLabel hRwLabel counter
    
    if isempty(counter)
        counter = 0;
        hWheels = zeros(1,4); hFlags = zeros(1,4); hTqFlags = zeros(1,2);
        hMotors = zeros(1,2); hSpokes = zeros(1,3); hCircles = zeros(1,4); hGdots = zeros(1,4);
        hSwLabel = 0.0; hRwLabel = 0.0;
        
        hFig = figure('Name', 'Vehicle Frame Telemetry', 'Color', 'w', 'Position', [950, 100, 750, 750]);
        hold on;
        
        plot([-1, 1, 1, -1, -1], [2, 2, -2, -2, 2], 'k', 'LineWidth', 2);
        hAxle = line([1, -1], [1.5, 1.5], 'Color', [0.2 0.2 0.2], 'LineWidth', 2);
        
        wheel_base = [-.2, .2, .2, -.2]; wheel_wid = [.4, .4, -.4, -.4];
        for i = 1:4; hWheels(i) = double(patch(0, 0, [0.3 0.3 0.3])); end
        
        m_b = [-.15, .15, .15, -.15]; m_w = [.2, .2, -.2, -.2];
        hMotors(1) = double(patch(m_b + 0.6, m_w - 1.5, [0.5 0.5 0.5]));
        hMotors(2) = double(patch(m_b - 0.6, m_w - 1.5, [0.5 0.5 0.5]));
        
        th_c = 0:0.1:2*pi;
        circle_x = cos(th_c); circle_y = sin(th_c);
        c_pos = [2.0, 2.3; -2.0, 2.3; 2.0, -2.3; -2.0, -2.3];
        for i = 1:4
            hCircles(i) = double(plot(c_pos(i,1) + 0.5*circle_x, c_pos(i,2) + 0.5*circle_y, 'Color', [0.6 0 0.6], 'LineStyle', '--', 'LineWidth', 1.2));
            hGdots(i) = double(plot(c_pos(i,1), c_pos(i,2), 'mo', 'MarkerFaceColor', 'm', 'MarkerSize', 5));
        end
        
        th = 0:0.1:2*pi;
        hSteer = double(plot(0.4*cos(th), 0.4*sin(th) + 0.5, 'k', 'LineWidth', 3));
        hSpokes(1) = double(line([0, 0], [0.5, 0.5], 'Color', 'k', 'LineWidth', 2.5));
        hSpokes(2) = double(line([0, 0], [0.5, 0.5], 'Color', 'k', 'LineWidth', 2.5));
        hSpokes(3) = double(line([0, 0], [0.5, 0.5], 'Color', 'k', 'LineWidth', 2.5));
        
        hPsiRef = double(quiver(0, 1.8, 0, 0.8, 'r', 'LineWidth', 2.5, 'MaxHeadSize', 2));
        hPsiAct = double(quiver(0, 1.8, 0, 0.8, 'b', 'LineWidth', 2.5, 'MaxHeadSize', 2));
        
        for i = 1:4; hFlags(i) = double(text(0, 0, '', 'FontSize', 8, 'BackgroundColor', [1 1 1 0.8], 'EdgeColor', 'k')); end
        hTqFlags(1) = double(text(0.6, -1.1, '', 'FontSize', 8, 'FontWeight', 'bold', 'HorizontalAlignment', 'center'));
        hTqFlags(2) = double(text(-0.6, -1.1, '', 'FontSize', 8, 'FontWeight', 'bold', 'HorizontalAlignment', 'center'));
        
        hSwLabel = double(text(0, 0, '', 'FontSize', 9, 'FontWeight', 'bold', 'HorizontalAlignment', 'center'));
        hRwLabel = double(text(0, 2.3, '', 'FontSize', 9, 'FontWeight', 'bold', 'HorizontalAlignment', 'center', 'Color', [0 0.5 0]));
        
        axis([-4.5 4.5 -4.5 4.5]); axis equal; grid on;
        title('Dynamics: Forces, Steering & Friction Circles');
    end
    counter = counter + 1;
    if mod(counter, 10) == 0
        R_delta = [cos(delta) -sin(delta); sin(delta) cos(delta)];
        w_orig = [-.2 .2 .2 -.2; .4 .4 -.4 -.4]; 
        w_rot = R_delta * w_orig;
        
        set(hWheels(1), 'XData', w_rot(1,:) + 1, 'YData', w_rot(2,:) + 1.5);
        set(hWheels(2), 'XData', w_rot(1,:) - 1, 'YData', w_rot(2,:) + 1.5);
        set(hWheels(3), 'XData', w_orig(1,:) + 1, 'YData', w_orig(2,:) - 1.5);
        set(hWheels(4), 'XData', w_orig(1,:) - 1, 'YData', w_orig(2,:) - 1.5);
        
        set(hAxle, 'XData', [mean(w_rot(1,:) + 1), mean(w_rot(1,:) - 1)], 'YData', [mean(w_rot(2,:) + 1.5), mean(w_rot(2,:) + 1.5)]);
        
        sw_a = delta * 14; 
        th_sw = (0:0.1:2*pi) + sw_a;
        set(hSteer, 'XData', 0.4*cos(th_sw), 'YData', 0.4*sin(th_sw) + 0.5);
        
        spk = [0, pi, 1.5*pi] + sw_a;
        for j=1:3; set(hSpokes(j), 'XData', [0, 0.4*cos(spk(j))], 'YData', [0.5, 0.5 + 0.4*sin(spk(j))]); end
        
        set(hSwLabel, 'Position', [0, 0.5], 'String', sprintf('SW: %.1f deg', sw_a * 180/pi));
        set(hRwLabel, 'String', sprintf('RW: %.1f deg', delta * 180/pi));
        
        psi_e = psi_ref - psi; 
        set(hPsiRef, 'UData', 0.8*sin(psi_e), 'VData', 0.8*cos(psi_e));
        set(hPsiAct, 'UData', 0, 'VData', 0.8);
        
        fb = [abs(Tf_f/2), abs(Tf_f/2), abs(Trl_f), abs(Trr_f)]; mu = 1.0;
        c_pos = [2.0, 2.3; -2.0, 2.3; 2.0, -2.3; -2.0, -2.3];
        th_c = 0:0.1:2*pi;
        
        % Convert rad/s to RPM
        rpm_vec = w_vec * (30 / pi);
        
        for i = 1:4
            if fb(i) > 5; set(hWheels(i), 'FaceColor', [0.8 0 0]); else set(hWheels(i), 'FaceColor', [0.3 0.3 0.3]); end
            F_max = max(100, mu * Fz(i));
            scale = 0.5 / 6000; 
            set(hCircles(i), 'XData', c_pos(i,1) + F_max*scale*cos(th_c), 'YData', c_pos(i,2) + F_max*scale*sin(th_c));
            set(hGdots(i), 'XData', c_pos(i,1) + Fy(i)*scale, 'YData', c_pos(i,2) + Fx(i)*scale);
        end
        
        mt = [Trl, Trr];
        for k = 1:2
            if mt(k) > 0.1; set(hMotors(k), 'FaceColor', [0 0.7 0]); elseif mt(k) < -0.1; set(hMotors(k), 'FaceColor', [0.7 0 0]); else set(hMotors(k), 'FaceColor', [0.5 0.5 0.5]); end
            set(hTqFlags(k), 'String', sprintf('Mot. Trq.\n%.1f Nm', mt(k)));
        end
        
        pos = [2.8, 1.5; -4.1, 1.5; 2.8, -1.5; -4.1, -1.5];
        for i = 1:4
            f_str = sprintf('Fx: %.0f\nFy: %.0f\nFz: %.0f\nFric: %.1f\nRPM: %.0f', Fx(i), Fy(i), Fz(i), fb(i), rpm_vec(i));
            set(hFlags(i), 'Position', [pos(i,1), pos(i,2)], 'String', f_str);
        end
        drawnow limitrate;
    end
end

== matlab function DLC_2a/Vehicle Control Unit (VCU)/MATLAB Function ==
  settings: updateMethod=DISCRETE
  data: delta_curr input; pedal input; T_rr_motor_raw output; vx_curr input; vy_curr input; r_curr input; kappa_ref input; Fz_f_total input; Fz_r_total input; Fz_rl input; Fz_rr input; SOC input; T_batt input; T_motor input; V_op parameter; K_scheduled parameter; T_rl_motor_raw output; T_rr_fric output; w_vec input; T_rl_fric output; T_f_fric output; Mz_cmd output; r_ref output
function [T_rr_motor_raw, T_rl_motor_raw, T_rr_fric, T_rl_fric, T_f_fric, Mz_cmd, r_ref] = vcu_allocator(delta_curr, pedal, vx_curr, vy_curr, r_curr, kappa_ref, Fz_f_total, Fz_r_total, Fz_rl, Fz_rr, SOC, T_batt, T_motor, V_op, K_scheduled, w_vec)


T_rr_motor_raw = 0.0;

T_rl_motor_raw = 0.0;

T_rr_fric = 0.0;

T_rl_fric = 0.0;

T_f_fric = 0.0;

Mz_cmd = 0.0;

Rw = 0.34; tw = 1.65; G = 10; mu_max = 1.2;


% --- Per-Motor Limits (Total System = 500 kW, 800 Nm) ---

P_motor_base = 250000; % 250 kW per motor

T_motor_max = 400; % 400 Nm per motor

T_fric_max_per_wheel = 3500;

% --------------------------------------------------------


% --- Battery and Thermal Derating ---

T_batt_cal = [-10, 0, 15, 45, 55, 60]; P_derate_batt_cal = [0, 0.5, 1.0, 1.0, 0.2, 0];

T_motor_cal = [30, 90, 110, 130, 150]; P_derate_motor_cal = [1.0, 1.0, 0.8, 0.2, 0];

SOC_vec = [0, 0.05, 0.15, 0.85, 0.95, 1.0];

P_derate_SOC_dis = [0, 0.1, 1.0, 1.0, 1.0, 1.0]; P_derate_SOC_chg = [1.0, 1.0, 1.0, 1.0, 0.1, 0];


derate_T_batt = interp1(T_batt_cal, P_derate_batt_cal, T_batt(1), 'linear', 0);

derate_T_mot = interp1(T_motor_cal, P_derate_motor_cal, T_motor(1), 'linear', 0);

derate_T_total = min(derate_T_batt, derate_T_mot);


derate_S_dis = interp1(SOC_vec, P_derate_SOC_dis, SOC(1), 'linear', 0);

derate_S_chg = interp1(SOC_vec, P_derate_SOC_chg, SOC(1), 'linear', 0);


P_avail_dis = P_motor_base * min(derate_T_total, derate_S_dis);

P_avail_chg = P_motor_base * min(derate_T_total, derate_S_chg);


vx_lqr = max(vx_curr(1), 5.0);


% --- Speed-based Torque Vectoring Blending (45 km/h to 50 km/h) ---

vx_kmh = vx_curr(1) * 3.6;

tv_blend_lower = 45.0;

tv_blend_upper = 50.0;


if vx_kmh >= tv_blend_upper

tv_blend = 1.0;

elseif vx_kmh <= tv_blend_lower

tv_blend = 0.0;

else

tv_blend = (vx_kmh - tv_blend_lower) / (tv_blend_upper - tv_blend_lower);

end


% --- LQR Yaw Moment Calculation ---

K_dyn_1 = interp1(V_op, K_scheduled(:,1), vx_lqr, 'linear', 'extrap');

K_dyn_2 = interp1(V_op, K_scheduled(:,2), vx_lqr, 'linear', 'extrap');


% =========================================================================

% 1. DYNAMIC ACKERMANN REFERENCE

% =========================================================================

L = 2.6; % Wheelbase

K_us = 0.0015; % Small understeer gradient (optional)

r_ref_raw = (vx_lqr * delta_curr(1)) / (L * (1 + K_us * vx_lqr^2));


% =========================================================================

% 2. PHYSICAL YAW RATE BOUNDING (The Jitter Fix)

% =========================================================================

g = 9.81;

% Calculate the absolute maximum yaw rate the tires can sustain

% based on current speed and track friction (r_max = mu * g / Vx)

% We use 0.95 as a safety margin to prevent fighting the TCS limiters.

r_max_phys = (mu_max * g * 0.95) / vx_lqr;


% Clamp the reference so the LQR never demands an impossible turn

r_ref = max(-r_max_phys, min(r_max_phys, r_ref_raw));

% =========================================================================

TV_Bite_Factor = 1;

vy_factor = 1;

Mz_req = tv_blend * -(vy_factor * K_dyn_1(1) * vy_curr(1) + TV_Bite_Factor * K_dyn_2(1) * (r_curr(1) - r_ref));

Mz_cmd = max(-2500, min(2500, Mz_req));


T_delta_wheel_raw = max(-1500, min(1500, (Mz_cmd * Rw) / tw));


% =========================================================================

% --- DYNAMIC MOTOR POWER LIMITS (Hyperbolic Torque Derating) ---

% =========================================================================

% Calculate actual motor speed from wheel speed (rad/s)

% w_vec = [w_fl, w_fr, w_rl, w_rr]

w_motor_rl = max(abs(w_vec(3) * G), 0.1); % Prevent div-by-zero at standstill

w_motor_rr = max(abs(w_vec(4) * G), 0.1);


% Power-limited torque curve: T_max = P_max / w

T_limit_rl_dis = P_avail_dis / w_motor_rl;

T_limit_rr_dis = P_avail_dis / w_motor_rr;

T_limit_rl_chg = P_avail_chg / w_motor_rl;

T_limit_rr_chg = P_avail_chg / w_motor_rr;


% Final motor bounds (Minimum of Inverter current limit and Power limit)

T_motor_lim_rl_dis = min(T_motor_max, T_limit_rl_dis);

T_motor_lim_rr_dis = min(T_motor_max, T_limit_rr_dis);


T_motor_lim_rl_chg = max(-T_motor_max, -T_limit_rl_chg);

T_motor_lim_rr_chg = max(-T_motor_max, -T_limit_rr_chg);

% =========================================================================


T_grip_lim_rl_wheel = mu_max * Fz_rl(1) * Rw * 0.90;

T_grip_lim_rr_wheel = mu_max * Fz_rr(1) * Rw * 0.90;


% Combine physical motor limits with dynamic grip limits

T_max_rl_motor = min(T_motor_lim_rl_dis, T_grip_lim_rl_wheel / G);

T_max_rr_motor = min(T_motor_lim_rr_dis, T_grip_lim_rr_wheel / G);

T_min_rl_motor = max(T_motor_lim_rl_chg, -T_grip_lim_rl_wheel / G);

T_min_rr_motor = max(T_motor_lim_rr_chg, -T_grip_lim_rr_wheel / G);


weight_rl = Fz_rl(1) / max(1, (Fz_rl(1) + Fz_rr(1)));

weight_rr = Fz_rr(1) / max(1, (Fz_rl(1) + Fz_rr(1)));


% --- DRIVE MODE ---

if pedal(1) >= 0

% Total requested drive torque, limited by combined max capabilities

T_req_total_motor = pedal(1) * (T_max_rl_motor + T_max_rr_motor);


T_rr_base_motor = T_req_total_motor * weight_rr;

T_rl_base_motor = T_req_total_motor * weight_rl;


T_rr_ideal = max(T_min_rr_motor, min(T_max_rr_motor, T_rr_base_motor + (T_delta_wheel_raw/G)));

T_rl_ideal = max(T_min_rl_motor, min(T_max_rl_motor, T_rl_base_motor - (T_delta_wheel_raw/G)));


% Traction Control (TCS)

v_hub_rl = max(vx_curr(1) - (tw/2)*r_curr(1), 1.0);

v_hub_rr = max(vx_curr(1) + (tw/2)*r_curr(1), 1.0);


kappa_rl = (w_vec(3)*Rw - v_hub_rl) / v_hub_rl;

kappa_rr = (w_vec(4)*Rw - v_hub_rr) / v_hub_rr;


slip_target = 0.10;

Kp_tcs = 1000;


if kappa_rl > slip_target

T_rl_ideal = max(0, T_rl_ideal - Kp_tcs * (kappa_rl - slip_target));

end

if kappa_rr > slip_target

T_rr_ideal = max(0, T_rr_ideal - Kp_tcs * (kappa_rr - slip_target));

end


T_rr_fric = 0; T_rl_fric = 0; T_f_fric = 0;


% --- BRAKE MODE ---

else

bias_f = 0.70;

total_grip_cap_wheel = mu_max * (Fz_f_total(1) + Fz_r_total(1)) * Rw * 0.90;

T_req_total_wheel = pedal(1) * total_grip_cap_wheel;


T_req_front_wheel = T_req_total_wheel * bias_f;

T_req_rear_wheel = T_req_total_wheel * (1 - bias_f);


T_f_fric = max(-mu_max * Fz_f_total(1) * Rw * 0.90, T_req_front_wheel);


T_base_rr = max(-(T_grip_lim_rr_wheel - abs(T_delta_wheel_raw)), T_req_rear_wheel * weight_rr);

T_base_rl = max(-(T_grip_lim_rl_wheel - abs(T_delta_wheel_raw)), T_req_rear_wheel * weight_rl);


T_rr_ideal_wheel = T_base_rr + T_delta_wheel_raw;

T_rl_ideal_wheel = T_base_rl - T_delta_wheel_raw;


% Anti-Lock Braking (ABS)

v_hub_fl = max(vx_curr(1) - (tw/2)*r_curr(1), 1.0);

v_hub_fr = max(vx_curr(1) + (tw/2)*r_curr(1), 1.0);

v_hub_rl = max(vx_curr(1) - (tw/2)*r_curr(1), 1.0);

v_hub_rr = max(vx_curr(1) + (tw/2)*r_curr(1), 1.0);


kappa_fl = (w_vec(1)*Rw - v_hub_fl) / v_hub_fl;

kappa_fr = (w_vec(2)*Rw - v_hub_fr) / v_hub_fr;

kappa_rl = (w_vec(3)*Rw - v_hub_rl) / v_hub_rl;

kappa_rr = (w_vec(4)*Rw - v_hub_rr) / v_hub_rr;


slip_limit_abs = -0.10;

Kp_abs = 5000;


worst_kappa_f = min(kappa_fl, kappa_fr);

if worst_kappa_f < slip_limit_abs

T_f_fric = min(0, T_f_fric - Kp_abs * (worst_kappa_f - slip_limit_abs));

end

if kappa_rl < slip_limit_abs

T_rl_ideal_wheel = min(0, T_rl_ideal_wheel - Kp_abs * (kappa_rl - slip_limit_abs));

end

if kappa_rr < slip_limit_abs

T_rr_ideal_wheel = min(0, T_rr_ideal_wheel - Kp_abs * (kappa_rr - slip_limit_abs));

end


T_rr_ideal = max(T_min_rr_motor, min(T_max_rr_motor, T_rr_ideal_wheel / G));

T_rl_ideal = max(T_min_rl_motor, min(T_max_rl_motor, T_rl_ideal_wheel / G));


T_rr_fric = max(-T_fric_max_per_wheel, min(0, T_rr_ideal_wheel - (T_rr_ideal * G)));

T_rl_fric = max(-T_fric_max_per_wheel, min(0, T_rl_ideal_wheel - (T_rl_ideal * G)));


if vx_curr(1) < 2.0

T_f_fric = 0; T_rr_fric = 0; T_rl_fric = 0;

T_rr_ideal = 0; T_rl_ideal = 0;

end

end


T_rr_motor_raw = T_rr_ideal;

T_rl_motor_raw = T_rl_ideal;

end
